simulink model "SMDFR_HTE_model"  (R2024b)
settings: Solver=ode15s  StartTime=1  StopTime=1200  FixedStep=0.01  RelTol=1e-3
model workspace (MAT data in the model file):
  ACS_lambda = 0.000161129786201
  A_cucl = 134.446
  A_cucl2 = 134.446
  A_cuocl = 213.991
  A_d = 217.647058824
  A_fw = [13.6 90 13.6]
  A_h = 217.647058824
  A_h2 = 217.647058824
  A_h20 = 18.015
  A_hcl = 36.458
  A_o = 32
  A_sg = 370
  A_wc = [10.9 103 10.9]
  C_c = 140.2
  C_cucl = 0.71
  C_cuocl = 1
  C_dst = 1996000
  C_h20 = 4.48
  C_hcl = 0.8
  C_hst = 1996000
  C_i0 = [429000000000000; 4.15e+15; 3.83e+15; 1.16e+16; 5.7e+15; 1.53e+15]
  C_o = 0.918
  Ce_i0 = [701000000000000; 5.88e+15; 3.36e+15; 5.09e+15; 820000000000000; 39600000000000]
  Cr = 0.00113148387097
  Cr_m = 8.769
  Cr_m_red = 4.3845
  Cr_red = 0.000565741935484
  D = 0.16
  DPB_lambda = 0.01
  EPB_lambda = 0.01
  E_d = 5
  E_e = 5
  E_h = 5
  E_hte = 5
  G_cucl = 44.778
  G_cucl2 = 44.778
  G_cuocl = 35.6355
  G_h2 = 32
  G_h20 = 10
  G_h20i = 10
  G_h20o = 7
  G_hcl = 12.1426
  G_o = 2.66
  G_s = 27000
  H_valve = 1
  Heat = [18744000 5970000 16956000]
  IPB_lambda = 0.01
  K_d = 500
  K_h = 500
  L = 6
  LOCA1 = 0
  LOCA2 = 0
  LOCA3 = 0
  LOCA4 = 0
  LOCA_p = 0.000161129786201
  LOCA_time = 300
  LOCA_times = [408 453 64 457 317 49 140 274 479 483 79 486 ... (4000 elements, 1000x4)]
  LOPC = 0
  LOPC_p = 0.1
  LOPC_times = [214 478 363 291 271 353 3 392 464 5 413 384 ... (1000 elements, 1000x1)]
  L_ACS = 0.01
  Lambda = 1.05e-06
  M_c = [219.9 7705 219.9]
  M_cucl0 = 44.778
  M_cucl20 = 44.778
  M_f = [307.7 1164 307.7]
  M_h20 = 8
  M_hcl0 = 12.1426
  M_w = [39.3 311 39.3]
  N = 1000
  N_0 = 15000000000000
  Nodes = 3
  P_0 = 100000000
  P_decomposition = 160
  P_hydro = 167
  Pb_acs : object (value not decoded)
  Pb_pipes : object (value not decoded)
  Pi_0 = [0.158 0.6899 0.152]
  Power_lambda = 0.01
  RPB_lambda = 0.01
  T_fw = 300
  T_hpi = 100
  T_st = 900
  Tbar_c0 = 1060
  Tbar_f0 = 1288
  Tc_in = 973
  Tin_c = 973
  Tin_f = 1300
  Tout_c = 1100
  Tout_f = 1300
  V_c = 160
  V_d = 160
  V_dst = 100
  V_h = 160
  V_h2 = 160
  V_hst = 100
  V_s = 100
  V_sg = 100
  age = 0
  ages = [0 50]
  alfa_c = -8.28e-06
  alfa_f = -0.000208
  alpha = 0.9926
  alpha_1 = 1
  alpha_2 = 1
  alpha_3 = 1
  alpha_4 = 1
  beta = 0.00302
  beta_i = [7.91e-05 0.000703 0.000504 0.00117 0.000457 0.00011]
  c_pc = [140.2 140.2 140.2]
  c_pf = [400 400 400]
  c_pw = [690 690 690]
  coolpipes = [2166 2166 0]
  d_c = 10187.40024
  d_dst = 3.14
  d_hst = 3.14
  d_st = 6.123
  demand = [0.661834040547 0.662423385196 0.661244695898 0.663602074493 0.660066006601 0.661244695898 0.662423385196 0.662423385196 0.662423385196 0.661244695898 0.661244695898 0.661244695898 ... (8761 elements, 8761x1)]
  diesel_lambda = 0.01
  eta = 0.4
  fail_threshold = 1244
  file = 'SMDFR_Parameters'
  fuelpipes = 1027
  h_dpo = 6801000
  h_fw = [6546 4305.1 7629.5]
  h_fw_st = 4386450
  h_hpo = 7159680
  h_in = 7000
  h_out = 1000
  h_st_in = 4386450
  h_wc = [27405.4 13833.4 32177.3]
  i = 1
  j = 1
  k_d = 2.7187
  k_e = 2.7187
  k_h = 0.005
  k_hte = 2.7187
  k_sg = 500
  lambda_c = 0.184
  lambda_e = 0.1
  lambda_i = [0.0127 0.03 0.11 0.319 1.18 7.02]
  leakage = 6.5
  mdot_c = [5550.5 5550.5 5550.5]
  mdot_c_value = 5550.5
  mdot_f = [327.7 327.7 327.7]
  mdot_f_value = 327.7
  model = 'SMDFR'
  mu = 50.9722799688
  mu_f = -20.9722799688
  mu_o = 30
  n = 0.45
  nsim = 1
  p_h20 = 40
  phi_tot = 3.61e+21
  rho = 7750
  rho_0 = 0.00111
  rhoex_value = 0
  sigma = 625
  sigma_c = 5
  sigma_f = 5.83095189485
  sigma_o = 3
  step = 0.1
  t = 0.008
  tau_c = 5.43
  tau_e = 10
  tr_fun : cfit (value not decoded)
  tsim = 500
  turbine_fun : cfit (value not decoded)
  v_rec = 4.16e-09
values from neighbouring files (symbols this model uses):
  ACS1_flow = 25    [Only_Inputs.m]    (also in Simulation_model.m; Simulation_model_complete.m; Simulation_model_hydrogen.m; Simulation_model_hydrogen_parallel.m)
  ACS1_response_time = randi(t_max_r_ACS-t_min_r_ACS)+t_min_r_ACS    [Failure_model.m]    (also in Failure_model_outputs.mat = 36; Only_Inputs.m = ACS1_response_time(indexes))
  ACS2_flow = 25    [Only_Inputs.m]    (also in Simulation_model.m; Simulation_model_complete.m; Simulation_model_hydrogen.m; Simulation_model_hydrogen_parallel.m)
  ACS2_response_time = randi(t_max_r_ACS-t_min_r_ACS)+t_min_r_ACS    [Failure_model.m]    (also in Failure_model_outputs.mat = 49; Only_Inputs.m = ACS2_response_time(indexes); Simulation_model_hydrogen_parallel.m = 0)
  ACS3_flow = 25    [Only_Inputs.m]    (also in Simulation_model.m; Simulation_model_complete.m; Simulation_model_hydrogen.m; Simulation_model_hydrogen_parallel.m)
  ACS3_response_time = randi(t_max_r_ACS-t_min_r_ACS)+t_min_r_ACS    [Failure_model.m]    (also in Failure_model_outputs.mat = 62; Only_Inputs.m = ACS3_response_time(indexes); Simulation_model_hydrogen_parallel.m = 0)
  ACS4_flow = 25    [Only_Inputs.m]    (also in Simulation_model.m; Simulation_model_complete.m; Simulation_model_hydrogen.m; Simulation_model_hydrogen_parallel.m)
  ACS4_response_time = randi(t_max_r_ACS-t_min_r_ACS)+t_min_r_ACS    [Failure_model.m]    (also in Failure_model_outputs.mat = 57; Only_Inputs.m = ACS4_response_time(indexes); Simulation_model_hydrogen_parallel.m = 0)
  ACS_1 = 821    [Failure_model_outputs.mat]    (also in Failure_sim.m = ACS_times(1); Only_Inputs.m = ACS_1(indexes))
  ACS_2 = 1010    [Failure_model_outputs.mat]    (also in Failure_sim.m = ACS_times(2); Only_Inputs.m = ACS_2(indexes); Simulation_model_hydrogen_parallel.m = 1)
  ACS_3 = 926    [Failure_model_outputs.mat]    (also in Failure_sim.m = ACS_times(3); Only_Inputs.m = ACS_3(indexes); Simulation_model_hydrogen_parallel.m = 1)
  ACS_4 = 80    [Failure_model_outputs.mat]    (also in Failure_sim.m = ACS_times(4); Only_Inputs.m = ACS_4(indexes); Simulation_model_hydrogen_parallel.m = 1)
  All_Outputs = 1    [Only_Inputs.m]    (also in Simulation_model.m = 0; Simulation_model_complete.m = 0; Simulation_model_hydrogen.m = 0; Simulation_model_hydrogen_parallel.m = 0)
  EDG1_response_time = randi(t_max_r_EDG-t_min_r_EDG)+t_min_r_EDG    [Failure_model.m]    (also in Failure_model_outputs.mat = 170; Only_Inputs.m = EDG1_response_time(indexes))
  EDG2_response_time = randi(t_max_r_EDG-t_min_r_EDG)+t_min_r_EDG    [Failure_model.m]    (also in Failure_model_outputs.mat = 133; Only_Inputs.m = EDG2_response_time(indexes); Simulation_model_hydrogen_parallel.m = 0)
  EDG_1 = 567    [Failure_model_outputs.mat]    (also in Only_Inputs.m = EDG_1(indexes))
  EDG_2 = 323    [Failure_model_outputs.mat]    (also in Only_Inputs.m = EDG_2(indexes); Simulation_model_hydrogen_parallel.m = 1)
  LHS = 0    [Failure_model_outputs.mat]    (also in Failure_sim.m = 60; Only_Inputs.m = LHS(indexes))
  LOCA1_time = 1200    [Failure_model_outputs.mat]    (also in Failure_sim.m = loca_times(1); Only_Inputs.m = LOCA1_time(indexes))
  LOCA2_time = 1200    [Failure_model_outputs.mat]    (also in Failure_sim.m = loca_times(2); Only_Inputs.m = LOCA2_time(indexes); Simulation_model_hydrogen_parallel.m)
  LOCA3_time = 39    [Failure_model_outputs.mat]    (also in Failure_sim.m = loca_times(3); Only_Inputs.m = LOCA3_time(indexes); Simulation_model_hydrogen_parallel.m = 1200)
  LOCA4_time = 18    [Failure_model_outputs.mat]    (also in Failure_sim.m = loca_times(4); Only_Inputs.m = LOCA4_time(indexes); Simulation_model_hydrogen_parallel.m = 1200)
  MSLB1 = 1200    [Failure_model_outputs.mat]    (also in Failure_sim.m = fix(randsample(x_loca, 1, true, lognorm_pdf)); Only_Inputs.m = MSLB1(indexes))
  MSLB2 = 1200    [Failure_model_outputs.mat]    (also in Failure_sim.m = fix(randsample(x_loca, 1, true, lognorm_pdf)); Only_Inputs.m = MSLB2(indexes); Simulation_model_hydrogen_parallel.m = 0)
  MSLB3 = 1200    [Failure_model_outputs.mat]    (also in Failure_sim.m = fix(randsample(x_loca, 1, true, lognorm_pdf)); Only_Inputs.m = MSLB3(indexes); Simulation_model_hydrogen_parallel.m = 0)
  MSLB4 = 1200    [Failure_model_outputs.mat]    (also in Failure_sim.m = fix(randsample(x_loca, 1, true, lognorm_pdf)); Only_Inputs.m = MSLB4(indexes); Simulation_model_hydrogen_parallel.m = 0)
  PDP11 = 1200    [Failure_model_outputs.mat]    (also in Failure_sim.m = pdp_times(1); Only_Inputs.m = PDP11(indexes))
  PDP11_response_time = randi(t_max_r_EDG-t_min_r_EDG)+t_min_r_EDG    [Failure_model.m]    (also in Failure_model_outputs.mat = 136; Only_Inputs.m = PDP11_response_time(indexes))
  PDP12 = 1200    [Failure_model_outputs.mat]    (also in Failure_sim.m = pdp_times(2); Only_Inputs.m = PDP12(indexes); Simulation_model_hydrogen_parallel.m = 0)
  PDP12_response_time = randi(t_max_r_EDG-t_min_r_EDG)+t_min_r_EDG    [Failure_model.m]    (also in Failure_model_outputs.mat = 119; Only_Inputs.m = PDP12_response_time(indexes); Simulation_model_hydrogen_parallel.m = 0)
  PDP21 = 1200    [Failure_model_outputs.mat]    (also in Failure_sim.m = pdp_times(3); Only_Inputs.m = PDP21(indexes); Simulation_model_hydrogen_parallel.m = 0)
  PDP21_response_time = randi(t_max_r_EDG-t_min_r_EDG)+t_min_r_EDG    [Failure_model.m]    (also in Failure_model_outputs.mat = 17; Only_Inputs.m = PDP21_response_time(indexes); Simulation_model_hydrogen_parallel.m = 0)
  PDP22 = 1200    [Failure_model_outputs.mat]    (also in Failure_sim.m = pdp_times(4); Only_Inputs.m = PDP22(indexes); Simulation_model_hydrogen_parallel.m = 0)
  PDP22_response_time = randi(t_max_r_EDG-t_min_r_EDG)+t_min_r_EDG    [Failure_model.m]    (also in Failure_model_outputs.mat = 120; Only_Inputs.m = PDP22_response_time(indexes); Simulation_model_hydrogen_parallel.m = 0)
  PDP31 = 1200    [Failure_model_outputs.mat]    (also in Failure_sim.m = pdp_times(5); Only_Inputs.m = PDP31(indexes); Simulation_model_hydrogen_parallel.m = 0)
  PDP31_response_time = randi(t_max_r_EDG-t_min_r_EDG)+t_min_r_EDG    [Failure_model.m]    (also in Failure_model_outputs.mat = 65; Only_Inputs.m = PDP31_response_time(indexes); Simulation_model_hydrogen_parallel.m = 0)
  PDP32 = 1200    [Failure_model_outputs.mat]    (also in Failure_sim.m = pdp_times(6); Only_Inputs.m = PDP32(indexes); Simulation_model_hydrogen_parallel.m = 0)
  PDP32_response_time = randi(t_max_r_EDG-t_min_r_EDG)+t_min_r_EDG    [Failure_model.m]    (also in Failure_model_outputs.mat = 28; Only_Inputs.m = PDP32_response_time(indexes); Simulation_model_hydrogen_parallel.m = 0)
  PDP41 = 1200    [Failure_model_outputs.mat]    (also in Failure_sim.m = pdp_times(7); Only_Inputs.m = PDP41(indexes); Simulation_model_hydrogen_parallel.m = 0)
  PDP41_response_time = randi(t_max_r_EDG-t_min_r_EDG)+t_min_r_EDG    [Failure_model.m]    (also in Failure_model_outputs.mat = 24; Only_Inputs.m = PDP41_response_time(indexes); Simulation_model_hydrogen_parallel.m = 0)
  PDP42 = 1200    [Failure_model_outputs.mat]    (also in Failure_sim.m = pdp_times(8); Only_Inputs.m = PDP42(indexes); Simulation_model_hydrogen_parallel.m = 0)
  PDP42_response_time = randi(t_max_r_EDG-t_min_r_EDG)+t_min_r_EDG    [Failure_model.m]    (also in Failure_model_outputs.mat = 164; Only_Inputs.m = PDP42_response_time(indexes); Simulation_model_hydrogen_parallel.m = 0)
  PGA = zeros(N,1)    [Crude_MC.m]    (also in Failure_model_outputs.mat = 0.3; Only_Inputs.m = PGA(indexes); Results.mat = [0.197697697698 0.158618618619 0.354014014014 0.1 0.1 0.4126; Simulation_model_hydrogen_parallel.m = 0)
  Power = 1200    [Failure_model_outputs.mat]    (also in Failure_sim.m = fix(randsample(x_loca, 1, true, lognorm_pdf)); Only_Inputs.m = Power(indexes))
  thermal_failure = 0    [Failure_model_outputs.mat]    (also in Failure_sim.m = 1; Only_Inputs.m = zeros(N,1); Simulation_model_hydrogen_parallel.m)
  thermal_failure_time = 1200    [Failure_model_outputs.mat]    (also in Failure_sim.m = 60; Only_Inputs.m = zeros(N,1); Simulation_model_hydrogen_parallel.m)
libraries: SMDFR_lib x8
(part 2 of 2)

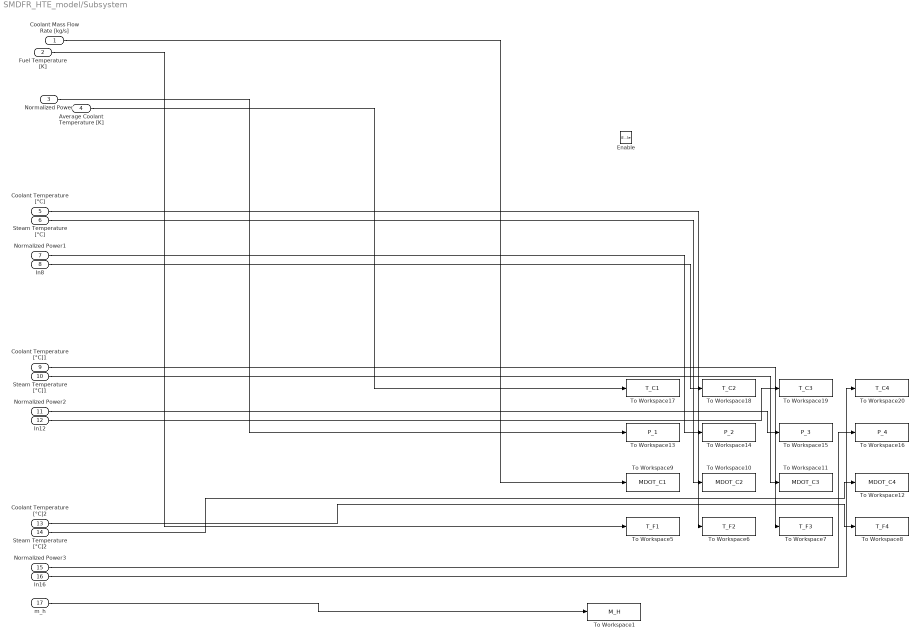
== system SMDFR_HTE_model/Subsystem ==
  Coolant Mass Flow Rate [kg/s] : Inport
  Fuel Temperature [K] : Inport  Port=2
  Normalized Power : Inport  Port=3
  Average Coolant Temperature [K] : Inport  Port=4
  Coolant Temperature [°C] : Inport  Port=5
  Steam Temperature [°C] : Inport  Port=6
  Normalized Power1 : Inport  Port=7
  In8 : Inport  Port=8
  Coolant Temperature [°C]1 : Inport  Port=9
  Steam Temperature [°C]1 : Inport  Port=10
  Normalized Power2 : Inport  Port=11
  In12 : Inport  Port=12
  Coolant Temperature [°C]2 : Inport  Port=13
  Steam Temperature [°C]2 : Inport  Port=14
  Normalized Power3 : Inport  Port=15
  In16 : Inport  Port=16
  m_h : Inport  Port=17
  Enable : EnablePort
  To Workspace1 : ToWorkspace  VariableName=M_H  SampleTime=1
  To Workspace10 : ToWorkspace  VariableName=MDOT_C2  SampleTime=1
  To Workspace11 : ToWorkspace  VariableName=MDOT_C3  SampleTime=1
  To Workspace12 : ToWorkspace  VariableName=MDOT_C4  SampleTime=1
  To Workspace13 : ToWorkspace  VariableName=P_1  SampleTime=1
  To Workspace14 : ToWorkspace  VariableName=P_2  SampleTime=1
  To Workspace15 : ToWorkspace  VariableName=P_3  SampleTime=1
  To Workspace16 : ToWorkspace  VariableName=P_4  SampleTime=1
  To Workspace17 : ToWorkspace  VariableName=T_C1  SampleTime=1
  To Workspace18 : ToWorkspace  VariableName=T_C2  SampleTime=1
  To Workspace19 : ToWorkspace  VariableName=T_C3  SampleTime=1
  To Workspace20 : ToWorkspace  VariableName=T_C4  SampleTime=1
  To Workspace5 : ToWorkspace  VariableName=T_F1  SampleTime=1
  To Workspace6 : ToWorkspace  VariableName=T_F2  SampleTime=1
  To Workspace7 : ToWorkspace  VariableName=T_F3  SampleTime=1
  To Workspace8 : ToWorkspace  VariableName=T_F4  SampleTime=1
  To Workspace9 : ToWorkspace  VariableName=MDOT_C1  SampleTime=1
  wires:
  Normalized Power/1 -> To Workspace13/1
  Coolant Temperature [°C]1/1 -> To Workspace7/1
  Coolant Mass Flow Rate [kg/s]/1 -> To Workspace9/1
  Average Coolant Temperature [K]/1 -> To Workspace17/1
  Fuel Temperature [K]/1 -> To Workspace5/1
  Coolant Temperature [°C]2/1 -> To Workspace8/1
  In12/1 -> To Workspace19/1
  In8/1 -> To Workspace18/1
  Coolant Temperature [°C]/1 -> To Workspace6/1
  Steam Temperature [°C]/1 -> To Workspace10/1
  In16/1 -> To Workspace20/1
  Normalized Power1/1 -> To Workspace14/1
  Steam Temperature [°C]1/1 -> To Workspace11/1
  Normalized Power2/1 -> To Workspace15/1
  Steam Temperature [°C]2/1 -> To Workspace12/1
  Normalized Power3/1 -> To Workspace16/1
  m_h/1 -> To Workspace1/1

== matlab function SMDFR_HTE_model/MATLAB Function8 ==
  data: M1_out output; time input; ACS1 input; ACS2 input; ACS3 input; ACS4 input; M2_out output; M3_out output; M4_out output; M1 input; M2 input; M3 input; M4 input; LOCA1_time parameter; LOCA2_time parameter; LOCA3_time parameter; LOCA4_time parameter; MSLB1 parameter; MSLB2 parameter; MSLB3 parameter; MSLB4 parameter
function [M1_out,M2_out,M3_out,M4_out] = fcn(time,ACS1,ACS2,ACS3,ACS4,M1,M2,M3,M4,LOCA1_time, LOCA2_time, LOCA3_time, LOCA4_time, MSLB1, MSLB2, MSLB3, MSLB4)
LOCA_fail=zeros(4,1);
increment = 0.1;
if LOCA1_time < time
    LOCA_fail(1) = 1;
end
if LOCA2_time < time
    LOCA_fail(2) = 1;
end
if LOCA3_time < time
    LOCA_fail(3) = 1;
end
if LOCA4_time < time
    LOCA_fail(4) = 1;
end

if sum(LOCA_fail)>0 && MSLB1>time && MSLB2>time && MSLB3>time && MSLB4>time
    M_out = LOCA_fail/sum(LOCA_fail)*(ACS1+ACS2+ACS3+ACS4);
    if mod(time,1)==0
        if M_out(1) > M1
            M1_out=min(M_out(1),M1+increment);
        else
            if M_out(1)<M1
                M1_out=max(M_out(1),M1-increment);
            else
                M1_out=M_out(1);
            end
        end
    else
        M1_out=M1;
    end
    if mod(time,1)==0
        if M_out(2) > M2
            M2_out=min(M_out(2),M2+increment);
        else
            if M_out(2)<M2
                M2_out=max(M_out(2),M2-increment);
            else
                M2_out=M_out(2);
            end
        end
    else
        M2_out=M2;
    end
    if mod(time,1)==0
        if M_out(3) > M3
            M3_out=min(M_out(3),M3+increment);
        else
            if M_out(3)<M3
                M3_out=max(M_out(3),M3-increment);
            else
                M3_out=M_out(3);
            end
        end
    else
        M3_out=M3;
    end
    if mod(time,1)==0
        if M_out(4) > M4
            M4_out=min(M_out(4),M4+increment);
        else
            if M_out(4)<M4
                M4_out=max(M_out(4),M4-increment);
            else
                M4_out=M_out(4);
            end
        end
    else
        M4_out=M4;
    end
else
    M_out=zeros(4,1);
    M1_out = M_out(1);
    M2_out = M_out(2);
    M3_out = M_out(3);
    M4_out = M_out(4);
end

factor=40*10;
if MSLB1<time
    M1_out = M1_out+(ACS1+ACS2+ACS3+ACS4)*factor;
end
if MSLB2<time
    M2_out = M2_out+(ACS1+ACS2+ACS3+ACS4)*factor;
end
if MSLB3<time
    M3_out = M3_out+(ACS1+ACS2+ACS3+ACS4)*factor;
end
if MSLB4<time
    M4_out = M4_out+(ACS1+ACS2+ACS3+ACS4)*factor;
end


end

== matlab function SMDFR_HTE_model/MATLAB Function ==
  data: t input; PDP1_fail output; MSLB1 parameter; PDP11_response_time parameter; PDP11 parameter; EDG input
function PDP1_fail = fcn(t,MSLB1, PDP11_response_time, PDP11, EDG)

if ((t<PDP11 || EDG) && t>(MSLB1+PDP11_response_time)) 
    PDP1_fail=0;
else
    PDP1_fail=1;
end

== matlab function SMDFR_HTE_model/MATLAB Function9 ==
  data: t input; PDP2_fail output; MSLB1 parameter; PDP12_response_time parameter; PDP12 parameter; EDG input
function PDP2_fail = fcn(t,MSLB1, PDP12_response_time, PDP12, EDG)

if ((t<PDP12 || EDG) && t>(MSLB1+PDP12_response_time)) 
    PDP2_fail=0;
else
    PDP2_fail=1;
end

== matlab function SMDFR_HTE_model/MATLAB Function10 ==
  data: t input; PDP1_fail output; MSLB2 parameter; PDP21_response_time parameter; PDP21 parameter; EDG input
function PDP1_fail = fcn(t,MSLB2, PDP21_response_time, PDP21, EDG)

if ((t<PDP21 || EDG) && t>(MSLB2+PDP21_response_time)) 
    PDP1_fail=0;
else
    PDP1_fail=1;
end

== matlab function SMDFR_HTE_model/MATLAB Function11 ==
  data: t input; PDP2_fail output; MSLB2 parameter; PDP22_response_time parameter; PDP22 parameter; EDG input
function PDP2_fail = fcn(t,MSLB2, PDP22_response_time, PDP22, EDG)

if ((t<PDP22 || EDG) && t>(MSLB2+PDP22_response_time)) 
    PDP2_fail=0;
else
    PDP2_fail=1;
end

== matlab function SMDFR_HTE_model/MATLAB Function12 ==
  data: t input; PDP1_fail output; MSLB4 parameter; PDP41_response_time parameter; PDP41 parameter; EDG input
function PDP1_fail = fcn(t,MSLB4, PDP41_response_time, PDP41, EDG)

if ((t<PDP41 || EDG) && t>(MSLB4+PDP41_response_time)) 
    PDP1_fail=0;
else
    PDP1_fail=1;
end

== matlab function SMDFR_HTE_model/MATLAB Function13 ==
  data: t input; PDP2_fail output; MSLB4 parameter; PDP42_response_time parameter; PDP42 parameter; EDG input
function PDP2_fail = fcn(t,MSLB4, PDP42_response_time, PDP42, EDG)

if ((t<PDP42 || EDG) && t>(MSLB4+PDP42_response_time)) 
    PDP2_fail=0;
else
    PDP2_fail=1;
end

== matlab function SMDFR_HTE_model/MATLAB Function14 ==
  data: t input; PDP1_fail output; MSLB3 parameter; PDP31_response_time parameter; PDP31 parameter; EDG input
function PDP1_fail = fcn(t,MSLB3, PDP31_response_time, PDP31, EDG)

if ((t<PDP31 || EDG) && t>(MSLB3+PDP31_response_time)) 
    PDP1_fail=0;
else
    PDP1_fail=1;
end

== matlab function SMDFR_HTE_model/MATLAB Function15 ==
  data: t input; PDP2_fail output; MSLB3 parameter; PDP32_response_time parameter; PDP32 parameter; EDG input
function PDP2_fail = fcn(t,MSLB3, PDP32_response_time, PDP32, EDG)

if ((t<PDP32 || EDG) && t>(MSLB3+PDP32_response_time)) 
    PDP2_fail=0;
else
    PDP2_fail=1;
end

== matlab function SMDFR_HTE_model/STEAM MASS FLOW RATE ==
  data: m_steam output; m_dot_c1 input; m_dot_c2 input; m_dot_c3 input; m_dot_c4 input; T_c1 input; T_c2 input; T_c3 input; T_c4 input; Tin_c1 input; Tin_c2 input; Tin_c3 input; Tin_c4 input
function m_steam = fcn(m_dot_c1,m_dot_c2,m_dot_c3,m_dot_c4,T_c1,T_c2,T_c3,T_c4,Tin_c1,Tin_c2,Tin_c3,Tin_c4)

cp = 140.2;
h_steam = 4.11*10^6;
h_coolant = 152920;

Q1 = m_dot_c1*cp*(T_c1-Tin_c1);
Q2 = m_dot_c2*cp*(T_c2-Tin_c2);
Q3 = m_dot_c3*cp*(T_c3-Tin_c3);
Q4 = m_dot_c4*cp*(T_c4-Tin_c4);

m_steam1 = Q1/(h_steam-h_coolant);
m_steam2 = Q2/(h_steam-h_coolant);
m_steam3 = Q3/(h_steam-h_coolant);
m_steam4 = Q4/(h_steam-h_coolant);

m_steam = m_steam1+m_steam2+m_steam3+m_steam4;

== matlab function SMDFR_HTE_model/HYDROGEN PRODUCTION ==
  data: m_steam input; m_h output
function m_h = fcn(m_steam)


T = 680; %°C
F = 96.485; % °C/mol
A = 0.0025; %m^2
r1 = 1; %assumption
r2 = 1e-5*5500; %assumption
p_catode = 1e-0; %assumption
p_anode = 1; %assumption
SU = 0.8;

N = 326; %number of fuel cells for 10 kW
N_real = N*500*10^6/10000;

E_max = 8.31*T/(4*F)*log(p_anode/p_catode);
i_max = 2*F*m_steam*55.51/(A*N_real);
V = (E_max+i_max*r1*SU)/(r1/r2*(1-SU)+1); %soe voltage

m_h = max(0,2.505*V-2.504);

== matlab function SMDFR_HTE_model/HYDROGEN FAILURES ==
  settings: updateMethod=DISCRETE
  data: m_dot input; Power output; PGA parameter; demand parameter; thermal_failure parameter; MSLB1 output; MSLB2 output; MSLB3 output; MSLB4 output; thermal_failure_time parameter; LHS parameter
function [Power,MSLB1,MSLB2,MSLB3,MSLB4] = fcn(m_dot,PGA, demand, thermal_failure, thermal_failure_time, LHS) 

Power = 1200;
MSLB1 = 1200;
MSLB2 = 1200;
MSLB3 = 1200;
MSLB4 = 1200;

tr_fun = @(x) min(1,1.54e-15.*x.^3-3.99e-10.*x.^2+3.52e-5.*x-0.0607);
sw_fun = @(x) min(1,1.6e-33.*x.^7-5.12e-28.*x.^6+6.36e-23.*x.^5-3.79e-18.*x.^4+1.14e-13.*x.^3-1.63e-9.*x.^2+1.62e-5.*x-0.0126);
turbine_fun = @(x) 7.61e-6.*x-0.06698;

distance = 250;

fragility_fun = @(PGA,alpha,beta_r,beta_u) normcdf(log(PGA/alpha)/sqrt(beta_r^2+beta_u^2));

%p_isolate = 0.9; %from HyRAM ESD
%alternative approach from "PERFORMANCE ASSESSMENT OF SAFETY BARRIERS IN LIQUID HYDROGEN BUNKERING OPERATIONS USING BAYESIAN NETWORK"
p_26 = 2.4e-2; p_27 = 1.17e-1; p_28 = 2.5e-1; p_29 = 4.77e-2; p_30 = 2.11E-2;
p_31 = 3.36e-1; p_32 = 4.42e-3; p_33 = 1.42e-3; p_34 = 2.52e-3; p_35 = 1.7e-3;
p_36 = 2.36e-3; p_37 = 1.54e-4; p_7 = 9.82e-3;
p_ESD = (1-(1-p_26)*(1-p_27)*(1-p_28))*(1-(1-p_29)*(1-p_30)*(1-p_31));
p_alarm_activation = (1-(1-p_34)*(1-(p_32+p_33-p_32*p_33)));
p_alarm = (1-(1-p_alarm_activation)*(1-(p_35+p_36-p_35*p_36)));
p_detection = p_alarm*(1-(1-p_29)*(1-p_7)*(1-p_37));
p_isolate = 1-(p_ESD+p_detection-p_ESD*p_detection);

%hydrogen release probability
%piping_f = fragility_fun(PGA2,4.8,0.35,0.5);
piping_f = fragility_fun(PGA,2.8,0.35,0.5);
LOP=0;
demand_p = demand(randi(8760));
LOP_thermal = 0;
LHS_thermal = 0;
if (rand()<piping_f && rand()<(1-p_isolate)) || thermal_failure  
    t = randi(120*60);
    d = 0.001+rand()*0.66;
    %Overpressure
    r=distance;
    m_dot=m_dot*demand_p;
    section = randi(5); %sampling where the leakage occurs to get op. conditions
    v = [3306,1899,2197,2230,2537]; %from python code CoolProp
    rho = [0.0385,0.111,0.139,0.217,0.3]; %from python code CoolProp
    rho = rho(section);
    v = v(section);
    m_dot_release = min(m_dot,v*rho*pi*d^2/4);
    m_H = m_dot_release*t;
    P_atm = 101325;
    E = 119*10^6*m_H*2;
    R = r*P_atm^(1/3)/E^(1/3);
    overpressure = 0.34.*R.^(-4/3)+0.062.*R.^(-2)+0.0033.*R.^(-3); %from "SANDIA - Final Report on Hydrogen Plant Hazards and Risk Analysis Supporting Hydrogen Plant Siting near Nuclear Power Plants"
    overpressure = overpressure*P_atm;
    
    %Power network fragility
    sw_f = min(1,max(0,sw_fun(overpressure)));
    tr_f = min(1,max(0,tr_fun(overpressure)));
    r1 = rand();
    r2 = rand();
    r3 = rand();
    
    if r1<sw_f || (r2<tr_f && r3<tr_f)
        LOP = 1;
    else
        LOP=0;
    end
    %from HyRAM ESD
    if m_dot_release < 0.125
        p_delayed_ign = 0.004;
    else
        if m_dot_release < 6.25
            p_delayed_ign = 0.027;
        else
            p_delayed_ign = 0.120;
        end
    end

    %alternative approach from "PERFORMANCE ASSESSMENT OF SAFETY BARRIERS IN LIQUID HYDROGEN BUNKERING OPERATIONS USING BAYESIAN NETWORK"
    %could implement fault tree
    %p_delayed_ign = (1.4e-4)/3;
    if rand()>p_delayed_ign
        LOP = 0;
    else
        if rand()<turbine_fun(overpressure)
            LHS = 1;
            LHS_explosion = 1;

            if thermal_failure
                LHS_thermal=1;
            end
        end

        if LOP
            if thermal_failure
                LOP_thermal=1;
            end
        end
    end
end
sigma = 1;
mu = log(10) + sigma^2;
x_loca = linspace(0.01, 500, 4000);
lognorm_pdf = lognpdf(x_loca, mu, sigma);
if LOP
    if LOP_thermal
        Power = thermal_failure_time;
    else
        Power = fix(randsample(x_loca, 1, true, lognorm_pdf));
    end
    LOP_hydrogen = 1;
else
    LOP_hydrogen = 0;
end

if LHS
    if LHS_thermal  
         MSLB1 = thermal_failure_time;
         MSLB2 = thermal_failure_time;
         MSLB3 = thermal_failure_time;
         MSLB4 = thermal_failure_time;
    else
        MSLB1 = fix(randsample(x_loca, 1, true, lognorm_pdf));
        MSLB2 = fix(randsample(x_loca, 1, true, lognorm_pdf));
        MSLB3 = fix(randsample(x_loca, 1, true, lognorm_pdf));
        MSLB4 = fix(randsample(x_loca, 1, true, lognorm_pdf));
    end
end

== matlab function SMDFR_HTE_model/MATLAB Function2 ==
  data: ACS input; y output; time input
function y = fcn(ACS,time)

if time > ACS
    y=0;
else
    y=1;
end

== matlab function SMDFR_HTE_model/MATLAB Function1 ==
  data: ACS input; y output; time input
function y = fcn(ACS,time)

if time > ACS
    y=0;
else
    y=1;
end

== matlab function SMDFR_HTE_model/MATLAB Function3 ==
  data: ACS input; y output; time input
function y = fcn(ACS,time)

if time > ACS
    y=0;
else
    y=1;
end

== matlab function SMDFR_HTE_model/MATLAB Function4 ==
  data: ACS input; y output; time input
function y= fcn(ACS,time)

if time > ACS
    y=0;
else
    y=1;
end

== matlab function SMDFR_HTE_model/MATLAB Function5 ==
  data: EDG input; LOP input; response_time input; EDG_working output; time input
function EDG_working = fcn(EDG,LOP, response_time, time)

if time > EDG
    EDG_working=0;
else
    if (time-LOP)>response_time
        EDG_working=1;
    else
        EDG_working=0;
    end
end

== matlab function SMDFR_HTE_model/MATLAB Function6 ==
  data: EDG input; LOP input; response_time input; EDG_working output; time input
function EDG_working = fcn(EDG,LOP, response_time, time)

if time > EDG
    EDG_working=0;
else
    if (time-LOP)>response_time
        EDG_working=1;
    else
        EDG_working=0;
    end
end

== matlab function SMDFR_HTE_model/MATLAB Function7 ==
  data: LOP input; Power_out output; time input
function Power_out = fcn(LOP,time)

if time > LOP
    Power_out=0;
else
    Power_out=1;
end
